simulink subsystem "PvtSubSys_VSM_LCKIE"  (R2020b)
settings: Solver=VariableStepAuto  StartTime=0.0  StopTime=10.0  RelTol=1e-3
values from neighbouring files (symbols this model uses):
  P_VSM_LCKIE_ClassInput = 0.0    [LCKIE.sldd]
  P_VSM_LCKIE_Laneoffset : value not decoded    [LCKIE.sldd]
  P_VSM_LCKIE_Laneoffset_BP : value not decoded    [LCKIE.sldd]
  P_VSM_LCKIE_LatC_DisOffofLanWidth : value not decoded    [LCKIE.sldd]
  P_VSM_LCKIE_LatC_DisOffofSpd : value not decoded    [LCKIE.sldd]
  P_VSM_LCKIE_LatC_DisSW = 0.0    [LCKIE.sldd]
  P_VSM_LCKIE_LatC_LanWidth : value not decoded    [LCKIE.sldd]
  P_VSM_LCKIE_LATC_LimitDis : value not decoded    [LCKIE.sldd]
  P_VSM_LCKIE_LATC_LimitDis_BP : value not decoded    [LCKIE.sldd]
  P_VSM_LCKIE_LatC_LimitDisEgoToObjSelt = 1.5    [LCKIE.sldd]
  P_VSM_LCKIE_LatC_LimitEgoToOppLane = 0.3    [LCKIE.sldd]
  P_VSM_LCKIE_LatC_maxLimitDisREToLane = 2.5    [LCKIE.sldd]
  P_VSM_LCKIE_LatC_minLimitDisREToLane = 1.2    [LCKIE.sldd]
  P_VSM_LCKIE_LatC_MoveEnableDis = 0.0    [LCKIE.sldd]
  P_VSM_LCKIE_LatC_RESafDis = 0.8    [LCKIE.sldd]
  P_VSM_LCKIE_LatC_SafeDisofLanWidth : value not decoded    [LCKIE.sldd]
  P_VSM_LCKIE_LatC_Spd : value not decoded    [LCKIE.sldd]
  P_VSM_LCKIE_LongC_d1 : value not decoded    [LCKIE.sldd]
  P_VSM_LCKIE_LongC_d2 : value not decoded    [LCKIE.sldd]
  P_VSM_LCKIE_LongC_DetaSpd : value not decoded    [LCKIE.sldd]
  P_VSM_LCKIE_LongC_DirecChangeDis = 20.0    [LCKIE.sldd]
  P_VSM_LCKIE_LongC_FleetOff = 80.0    [LCKIE.sldd]
  P_VSM_LCKIE_LongC_maxDis = 80.0    [LCKIE.sldd]
  P_VSM_LCKIE_LongC_minDis = 50.0    [LCKIE.sldd]
  P_VSM_LCKIE_LongC_ShutDownLongDis = -25.0    [LCKIE.sldd]
  P_VSM_LCKIE_LongC_ShutDownTTC = -4.0    [LCKIE.sldd]
  P_VSM_LCKIE_LongC_Spd : value not decoded    [LCKIE.sldd]
  P_VSM_LCKIE_LongC_toff = 10.0    [LCKIE.sldd]
  P_VSM_LCKIE_OFC_ActDis = 10.0    [LCKIE.sldd]
  P_VSM_LCKIE_OFC_DownDis = 10.0    [LCKIE.sldd]
  P_VSM_LCKIE_OFC_DownTTC = 5.0    [LCKIE.sldd]
  P_VSM_LCKIE_OFC_SafDis = 10.0    [LCKIE.sldd]
  P_VSM_LCKIE_OFC_Toff = 3.0    [LCKIE.sldd]
  P_VSM_LCKIE_ORC_LatDis = 1.8    [LCKIE.sldd]
  P_VSM_LCKIE_ORC_LimitDis1 = -30.0    [LCKIE.sldd]
  P_VSM_LCKIE_ORC_LimitDis2 = -10.0    [LCKIE.sldd]
  P_VSM_LCKIE_ORC_LimitTTC = 10.0    [LCKIE.sldd]
  P_VSM_LCKIE_ORC_LowSpd = -5.0    [LCKIE.sldd]
  P_VSM_LCKIE_POC_Delaytime : value not decoded    [LCKIE.sldd]
  P_VSM_LCKIE_POC_detaSpd : value not decoded    [LCKIE.sldd]
  P_VSM_LCKIE_POC_LimitDis = -15.0    [LCKIE.sldd]
  P_VSM_LCKIE_POC_LimitTTC = 2.0    [LCKIE.sldd]
  P_VSM_LCKIE_State_CurveMax = 0.005    [LCKIE.sldd]
  P_VSM_LCKIE_State_CurveMin = 0.0055555555555555558    [LCKIE.sldd]
  P_VSM_LCKIE_State_detaspd = 1.39    [LCKIE.sldd]
  P_VSM_LCKIE_State_detaspd_enable = 1.0    [LCKIE.sldd]
  P_VSM_LCKIE_State_DriverInputTrqValue_enable = 1.0    [LCKIE.sldd]
  P_VSM_LCKIE_State_ELKObjClc = 1.0    [LCKIE.sldd]
  P_VSM_LCKIE_State_HWASts_disable = 1.0    [LCKIE.sldd]
  P_VSM_LCKIE_State_IEObjClc = 1.0    [LCKIE.sldd]
  P_VSM_LCKIE_State_IFVReady = 1.0    [LCKIE.sldd]
  P_VSM_LCKIE_State_lamb_enable = 1.0    [LCKIE.sldd]
  P_VSM_LCKIE_State_Lanecurve_enable = 1.0    [LCKIE.sldd]
  P_VSM_LCKIE_State_LaneWidth_enable = 1.0    [LCKIE.sldd]
  P_VSM_LCKIE_State_Off2on = 3.0    [LCKIE.sldd]
  P_VSM_LCKIE_State_OppObjClc = 1.0    [LCKIE.sldd]
  P_VSM_LCKIE_STATE_ORCObjenable = 0.0    [LCKIE.sldd]
  P_VSM_LCKIE_State_Vehspeed_enable = 1.0    [LCKIE.sldd]
  P_VSM_LCKIE_State_wiper_enable = 1.0    [LCKIE.sldd]
  P_VSM_LCKIE_tcycle = 0.02    [LCKIE.sldd]
undefined symbols (not defined in the file or in its folder): P_Global_Vehicle_Length_m, P_Global_VehicleWidthMin_m, P_VSM_LSMC_SampleTime, STATE
libraries: simulink x62
(part 2 of 5)

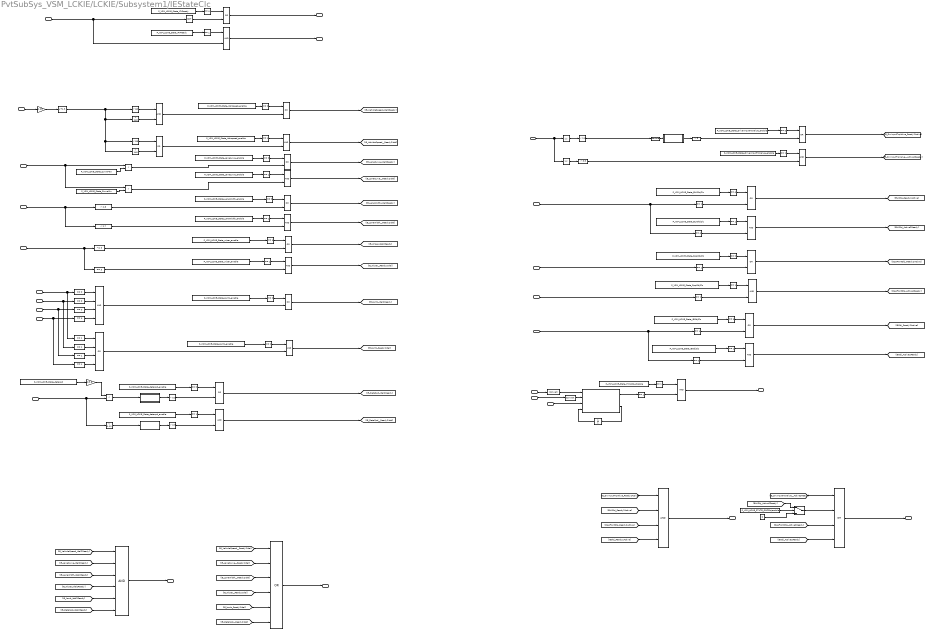
== system PvtSubSys_VSM_LCKIE/LCKIE/Subsystem1/IEStateClc ==
  note: IDEL2READY
  note: READY2ACTIVE
  LaneCurve : Inport
  LaneChange : Inport  Port=2
  OS_Roadwidth : Inport  Port=3
  OS_DetaSpdSelect : Inport  Port=4
  ORC_Clc : Inport  Port=5
  OFC_Ready : Inport  Port=6
  IEObj_Clc : Inport  Port=7
  OFC_Fail : Inport  Port=8
  canABSVehicleSpd : Inport  Port=9
  canBCMWiperSwitchSts : Inport  Port=10
  canBCMHighBeamSts : Inport  Port=11
  canBCMLowBeamSts : Inport  Port=12
  canBCMRearFogLmpSts : Inport  Port=13
  canBCMFrontFogLmpSts : Inport  Port=14
  EPS_DrvInputTrqValue3 : Inport  Port=15
  HWASts : Inport  Port=16
  IFC_Failsafe : Inport  Port=17
  LCKSts : Inport  Port=18
  Abs14 : Abs
  Abs5 : Abs
  Bias : Bias  Bias=1.3
  Compare To Constant1 : simulink/Logic and Bit Operations/Compare To Constant  relop=>  const=60  OutDataTypeStr=boolean
  Compare To Constant{2,7,9..11,14,17..18,23,28..29,33,42..46,48,90,113,182} (21 alike) : simulink/Logic and Bit Operations/Compare To Constant  relop===  const=1  OutDataTypeStr=boolean
  Compare To Constant{8,15..16,19..20,25,30,32,108,124,131..132,137..140,148} (17 alike) : simulink/Logic and Bit Operations/Compare To Constant  relop===  const=0  OutDataTypeStr=boolean
  Compare To Constant111 : simulink/Logic and Bit Operations/Compare To Constant  relop=<  const=55  OutDataTypeStr=boolean
  Compare To Constant112 : simulink/Logic and Bit Operations/Compare To Constant  relop=>  const=145  OutDataTypeStr=boolean
  Compare To Constant12 : simulink/Logic and Bit Operations/Compare To Constant  relop=<  const=-1.12  OutDataTypeStr=boolean
  Compare To Constant13 : simulink/Logic and Bit Operations/Compare To Constant  relop=<  const=2.5  OutDataTypeStr=boolean
  Compare To Constant145 : simulink/Logic and Bit Operations/Compare To Constant  relop=~=  const=3  OutDataTypeStr=boolean
  Compare To Constant21 : simulink/Logic and Bit Operations/Compare To Constant  relop=<  const=140  OutDataTypeStr=boolean
  Compare To Constant24 : simulink/Logic and Bit Operations/Compare To Constant  relop=>  const=0.5  OutDataTypeStr=boolean
  Compare To Constant26 : simulink/Logic and Bit Operations/Compare To Constant  relop=>  const=2.8  OutDataTypeStr=boolean
  Compare To Constant27 : simulink/Logic and Bit Operations/Compare To Constant  relop=<  const=2.7  OutDataTypeStr=boolean
  Compare To Constant3 : simulink/Logic and Bit Operations/Compare To Constant  relop=>  const=0.5  OutDataTypeStr=boolean
  Compare To Constant47 : simulink/Logic and Bit Operations/Compare To Constant  relop===  const=3  OutDataTypeStr=boolean
  Compare To Constant91 : simulink/Logic and Bit Operations/Compare To Constant  relop=>  const=3.5  OutDataTypeStr=boolean
  Compare To Constant31 : simulink/Logic and Bit Operations/Compare To Constant  relop=>  const=3  OutDataTypeStr=boolean
  Constant : Constant  Value=P_VSM_LCKIE_State_CurveMax
  Constant1 : Constant  Value=P_VSM_LCKIE_State_CurveMin
  Constant14 : Constant  Value=P_VSM_LCKIE_State_OppObjClc
  Constant15 : Constant  Value=P_VSM_LCKIE_State_IEObjClc
  Constant2 : Constant  Value=P_VSM_LCKIE_State_ELKObjClc
  Constant3 : Constant  Value=P_VSM_LCKIE_STATE_ORCObjenable
  Constant4 : Constant  Value=P_VSM_LCKIE_State_IEObjClc
  Constant5 : Constant  Value=0  OutDataTypeStr=boolean
  Constant8 : Constant  Value=P_VSM_LCKIE_State_ELKObjClc
  Constant9 : Constant  Value=P_VSM_LCKIE_State_OppObjClc
  Data Type Conversion : DataTypeConversion
  Data Type Conversion1 : DataTypeConversion
  Data Type Conversion15 : DataTypeConversion  OutDataTypeStr=double
  Gain : Gain  Gain=1/3.6
  Gain2 : Gain  Gain=1.03
  Logical Operator{1,4..5,9,11..13,17..18,21,49,60,64} (13 alike) : Logic  AllPortsSameDT=off  OutDataTypeStr=boolean
  Logical Operator{6..8,10,20,36,57,59,69,82..83,109} (12 alike) : Logic  Operator=OR  AllPortsSameDT=off  OutDataTypeStr=boolean
  Logical Operator101 : Logic  Operator=NOT  AllPortsSameDT=off  OutDataTypeStr=boolean
  Logical Operator14 : Logic  Inputs=6  AllPortsSameDT=off  OutDataTypeStr=boolean
  Logical Operator15 : Logic  Operator=OR  Inputs=6  AllPortsSameDT=off  OutDataTypeStr=boolean
  Logical Operator16 : Logic  Inputs=4  AllPortsSameDT=off  OutDataTypeStr=boolean
  Logical Operator19 : Logic  Operator=OR  Inputs=4  AllPortsSameDT=off  OutDataTypeStr=boolean
  Logical Operator22 : Logic  Operator=OR  Inputs=4  AllPortsSameDT=off  OutDataTypeStr=boolean
  Logical Operator89 : Logic  Inputs=4  AllPortsSameDT=off  OutDataTypeStr=boolean
  MATLAB Function1 : MATLAB Function  TreatAsAtomicUnit=on
  Relational Operator : RelationalOperator  Operator=<  OutDataTypeStr=boolean  RndMeth=Simplest
  Relational Operator1 : RelationalOperator  Operator=<  OutDataTypeStr=boolean  RndMeth=Simplest
  Relational Operator2 : RelationalOperator  Operator=>  OutDataTypeStr=boolean  RndMeth=Simplest
  Subsystem1 : Subsystem  mask{Ts=P_VSM_LSMC_SampleTime, Max=10}
      mask prompts: Ts "Sample Time:"; Max "Max Limit:"
      mask Display:
      | Ts=get_param(gcb,'Ts');
      | Max=get_param(gcb,'Max');
      | disp(['Ts:' Ts '\n' 'Max:' Max ]);
  Subsystem12 : Subsystem  mask{Ts=P_VSM_LSMC_SampleTime, Max=10}
      mask prompts: Ts "Sample Time:"; Max "Max Limit:"
      mask Display:
      | Ts=get_param(gcb,'Ts');
      | Max=get_param(gcb,'Max');
      | disp(['Ts:' Ts '\n' 'Max:' Max ]);
  Subsystem4 : Subsystem  mask{Ts=P_VSM_LSMC_SampleTime, Max=10}
      mask prompts: Ts "Sample Time:"; Max "Max Limit:"
      mask Display:
      | Ts=get_param(gcb,'Ts');
      | Max=get_param(gcb,'Max');
      | disp(['Ts:' Ts '\n' 'Max:' Max ]);
  Switch : Switch  Criteria=u2 > Threshold
  Unit Delay2 : UnitDelay  SampleTime=-1  HasFrameUpgradeWarning=on
  param_1 : Constant  Value=P_VSM_LCKIE_State_detaspd_enable
  param_14 : Constant  Value=P_VSM_LCKIE_State_wiper_enable
  param_15 : Constant  Value=P_VSM_LCKIE_State_lamb_enable
  param_16 : Constant  Value=P_VSM_LCKIE_State_Lanecurve_enable
  param_17 : Constant  Value=P_VSM_LCKIE_State_LaneWidth_enable
  param_2 : Constant  Value=P_VSM_LCKIE_State_detaspd_enable
  param_3 : Constant  Value=P_VSM_LCKIE_State_HWASts_disable
  param_31 : Constant  Value=P_VSM_LCKIE_State_Vehspeed_enable
  param_35 : Constant  Value=P_VSM_LCKIE_State_DriverInputTrqValue_enable
  param_4 : Constant  Value=P_VSM_LCKIE_State_Vehspeed_enable
  param_40 : Constant  Value=P_VSM_LCKIE_State_LaneWidth_enable
  param_45 : Constant  Value=P_VSM_LCKIE_State_wiper_enable
  param_46 : Constant  Value=P_VSM_LCKIE_State_lamb_enable
  param_5 : Constant  Value=P_VSM_LCKIE_State_detaspd
  param_6 : Constant  Value=P_VSM_LCKIE_State_IFVReady
  param_67 : Constant  Value=P_VSM_LCKIE_State_IFVReady
  param_7 : Constant  Value=P_VSM_LCKIE_State_DriverInputTrqValue_enable
  param_9 : Constant  Value=P_VSM_LCKIE_State_Lanecurve_enable
  IFVReady : Outport
  IFVFail : Outport  Port=2
  IE_Idel2Ready : Outport  Port=3
  IE_Ready2Idel : Outport  Port=4
  IE__Ready2Active : Outport  Port=5
  IE__Active2Ready : Outport  Port=6
  HWAReady : Outport  Port=7
  wires:
  [ELKObj_Active2Ready] -> Switch/1
  [OppFrontObj_Active2Ready] -> Logical Operator22/3
  [IEObj_Active2Ready] -> Logical Operator22/4
  [IE_DrvInputTrqValue__Active2Ready] -> Logical Operator22/1
  Logical Operator22/1 -> IE__Active2Ready/1  "VSM_LCKIE_State_Active2Ready"
  Logical Operator16/1 -> IE__Ready2Active/1  "VSM_LCKIE_State_Ready2Active"
  [IEObj_Ready2Active] -> Logical Operator16/4
  [OppFrontObj_Ready2Active] -> Logical Operator16/3
  [ELKObj_Ready2Active] -> Logical Operator16/2
  [IE_DrvInputTrqValue_Ready2Active] -> Logical Operator16/1
  Logical Operator15/1 -> IE_Ready2Idel/1  "VSM_LCKIE_State_Ready2Idel"
  [IE_DetaSpd__Ready2Idel] -> Logical Operator15/6
  [IE_lamb_Ready2Idel] -> Logical Operator15/5
  [IE_Wiper__Ready2Idel] -> Logical Operator15/4
  [IE_LaneWidth__Ready2Idel] -> Logical Operator15/3
  [IE_LaneCurve__Ready2Idel] -> Logical Operator15/2
  [IE_VehicleSpeed__Ready2Idel] -> Logical Operator15/1
  Logical Operator14/1 -> IE_Idel2Ready/1  "VSM_LCKIE_State_Idel2Ready"
  [IE_DetaSpd_Idel2Ready] -> Logical Operator14/6
  [IE_lamb_Idel2Ready] -> Logical Operator14/5
  [IE_Wiper_Idel2Ready] -> Logical Operator14/4
  [IE_LaneWidth_Idel2Ready] -> Logical Operator14/3
  [IE_LaneCurve_Idel2Ready] -> Logical Operator14/2
  [IE_VehicleSpeed_Idel2Ready] -> Logical Operator14/1
  Gain/1 -> Relational Operator/1
  param_5/1 -> Gain/1
  OFC_Fail/1 -> Compare To Constant11/1
  Compare To Constant9/1 -> Logical Operator12/1
  Constant8/1 -> Compare To Constant33/1
  Constant4/1 -> Compare To Constant16/1
  Logical Operator6/1 -> [ELKObj_Ready2Active]  "VSM_LCKIE_State_ELKObj_Ready2Active"
  Logical Operator10/1 -> [OppFrontObj_Ready2Active]  "VSM_LCKIE_State_OppFrontObj_Ready2Active"
  Compare To Constant18/1 -> Logical Operator6/2
  Constant15/1 -> Compare To Constant17/1
  IEObj_Clc/1 -> Compare To Constant29/1, Compare To Constant30/1
  Constant9/1 -> Compare To Constant9/1
  Logical Operator7/1 -> [IEObj_Ready2Active]  "VSM_LCKIE_State_IEObj_Ready2Active"
  Logical Operator13/1 -> [IEObj_Active2Ready]  "VSM_LCKIE_State_IEObj_Active2Ready"
  Compare To Constant8/1 -> Logical Operator10/1
  Compare To Constant11/1 -> Logical Operator12/2
  ORC_Clc/1 -> Compare To Constant18/1, Compare To Constant19/1
  Compare To Constant10/1 -> Logical Operator10/2
  Compare To Constant32/1 -> Logical Operator6/1
  Compare To Constant19/1 -> Logical Operator9/2
  Constant2/1 -> Compare To Constant32/1
  Compare To Constant30/1 -> Logical Operator13/2
  Compare To Constant29/1 -> Logical Operator7/2
  Compare To Constant16/1 -> Logical Operator7/1
  Compare To Constant17/1 -> Logical Operator13/1
  Logical Operator12/1 -> [OppFrontObj_Active2Ready]  "VSM_LCKIE_State_OppFrontObj_Active2Ready"
  OFC_Ready/1 -> Compare To Constant10/1
  Constant14/1 -> Compare To Constant8/1
  Logical Operator9/1 -> [ELKObj_Active2Ready]  "VSM_LCKIE_State_ELKObj_Active2Ready"
  Compare To Constant33/1 -> Logical Operator9/1
  IFC_Failsafe/1 -> Logical Operator101/1, Logical Operator5/2
  Compare To Constant148/1 -> Logical Operator109/1
  Logical Operator5/1 -> IFVFail/1  "VSM_LCKIE_State_IFVFail"
  Logical Operator109/1 -> IFVReady/1  "VSM_LCKIE_State_IFVReady"
  param_67/1 -> Compare To Constant182/1
  param_6/1 -> Compare To Constant148/1
  Compare To Constant182/1 -> Logical Operator5/1
  Logical Operator101/1 -> Logical Operator109/2
  Data Type Conversion15/1 -> Subsystem12/1(In1)
  Compare To Constant90/1 -> Logical Operator49/1
  Compare To Constant124/1 -> Logical Operator69/1
  EPS_DrvInputTrqValue3/1 -> Abs5/1, Abs14/1
  Compare To Constant13/1 -> Data Type Conversion15/1
  Compare To Constant31/1 -> Logical Operator69/2
  Abs14/1 -> Compare To Constant91/1
  Logical Operator49/1 -> [IE_DrvInputTrqValue__Active2Ready]  "VSM_LCKIE_State_DrvInputTrqValue_Active2Ready"
  Subsystem12/1(Out1) -> Compare To Constant31/1
  Logical Operator69/1 -> [IE_DrvInputTrqValue_Ready2Active]  "VSM_LCKIE_State_DrvInputTrqValue_Ready2Active"
  Abs5/1 -> Compare To Constant13/1
  param_35/1 -> Compare To Constant90/1
  Compare To Constant91/1 -> Logical Operator49/2
  param_7/1 -> Compare To Constant124/1
  HWASts/1 -> Data Type Conversion/1
  param_3/1 -> Compare To Constant7/1
  Compare To Constant7/1 -> Logical Operator4/1
  Logical Operator4/1 -> HWAReady/1  "VSM_LCKIE_State_HWASts_Ready2Active"
  Logical Operator1/1 -> [IE_DetaSpd__Ready2Idel]  "VSM_LCKIE_State_detaspd_Ready2Idel"
  Compare To Constant12/1 -> Subsystem4/1(In1)
  Compare To Constant2/1 -> Logical Operator1/1
  param_2/1 -> Compare To Constant2/1
  Compare To Constant3/1 -> Logical Operator1/2
  Subsystem4/1(Out1) -> Compare To Constant3/1
  Subsystem1/1(Out1) -> Compare To Constant24/1
  Compare To Constant24/1 -> Logical Operator8/2
  param_1/1 -> Compare To Constant15/1
  Relational Operator/1 -> Subsystem1/1(In1)
  Logical Operator8/1 -> [IE_DetaSpd_Idel2Ready]  "VSM_LCKIE_State_detaspd_Idel2Ready"
  Compare To Constant15/1 -> Logical Operator8/1
  OS_DetaSpdSelect/1 -> Compare To Constant12/1, Relational Operator/2
  Compare To Constant131/1 -> Logical Operator82/1
  param_45/1 -> Compare To Constant131/1
  Logical Operator83/1 -> [IE_lamb_Idel2Ready]  "VSM_LCKIE_State_lamb_Idel2Ready"
  Compare To Constant139/1 -> Logical Operator89/3
  Logical Operator82/1 -> [IE_Wiper_Idel2Ready]  "VSM_LCKIE_State_wiper_Idel2Ready"
  canBCMLowBeamSts/1 -> Compare To Constant138/1, Compare To Constant44/1
  canBCMWiperSwitchSts/1 -> Compare To Constant145/1, Compare To Constant47/1
  canBCMHighBeamSts/1 -> Compare To Constant137/1, Compare To Constant42/1
  param_46/1 -> Compare To Constant132/1
  Logical Operator89/1 -> Logical Operator83/2
  Compare To Constant137/1 -> Logical Operator89/1
  canBCMFrontFogLmpSts/1 -> Compare To Constant140/1, Compare To Constant46/1
  Compare To Constant140/1 -> Logical Operator89/4
  Compare To Constant145/1 -> Logical Operator82/2
  Compare To Constant132/1 -> Logical Operator83/1
  canBCMRearFogLmpSts/1 -> Compare To Constant139/1, Compare To Constant45/1
  Compare To Constant138/1 -> Logical Operator89/2
  Compare To Constant27/1 -> Logical Operator21/2
  Logical Operator21/1 -> [IE_LaneWidth__Ready2Idel]  "VSM_LCKIE_State_LaneWidth_Ready2Idel"
  Compare To Constant28/1 -> Logical Operator21/1
  param_17/1 -> Compare To Constant28/1
  Compare To Constant26/1 -> Logical Operator20/2
  param_40/1 -> Compare To Constant25/1
  Logical Operator20/1 -> [IE_LaneWidth_Idel2Ready]  "VSM_LCKIE_State_LaneWidth_Idel2Ready"
  Compare To Constant25/1 -> Logical Operator20/1
  OS_Roadwidth/1 -> Compare To Constant26/1, Compare To Constant27/1
  Compare To Constant23/1 -> Logical Operator11/1
  Relational Operator2/1 -> Logical Operator11/2
  param_16/1 -> Compare To Constant23/1
  Logical Operator11/1 -> [IE_LaneCurve__Ready2Idel]  "VSM_LCKIE_State_Lanecurve_Ready2Idel"
  Logical Operator36/1 -> [IE_LaneCurve_Idel2Ready]  "VSM_LCKIE_State_Lanecurve_Idel2Ready"
  param_9/1 -> Compare To Constant108/1
  LaneCurve/1 -> Relational Operator2/1, Relational Operator1/1
  Relational Operator1/1 -> Logical Operator36/2
  Compare To Constant108/1 -> Logical Operator36/1
  Compare To Constant21/1 -> Logical Operator60/2
  Bias/1 -> Compare To Constant112/1, Compare To Constant111/1, Compare To Constant21/1, Compare To Constant1/1
  param_31/1 -> Compare To Constant20/1
  param_4/1 -> Compare To Constant113/1
  Compare To Constant112/1 -> Logical Operator57/2
  Logical Operator59/1 -> [IE_VehicleSpeed_Idel2Ready]  "VSM_LCKIE_State_Vehspeed_Idel2Ready"
  Logical Operator57/1 -> Logical Operator64/2
  Logical Operator64/1 -> [IE_VehicleSpeed__Ready2Idel]  "VSM_LCKIE_State_Vehspeed_Ready2Idel"
  Compare To Constant20/1 -> Logical Operator59/1
  Compare To Constant113/1 -> Logical Operator64/1
  Gain2/1 -> Bias/1
  canABSVehicleSpd/1 -> Gain2/1
  Compare To Constant1/1 -> Logical Operator60/1
  Logical Operator60/1 -> Logical Operator59/2
  Compare To Constant111/1 -> Logical Operator57/1
  Compare To Constant45/1 -> Logical Operator19/3
  param_15/1 -> Compare To Constant43/1
  Compare To Constant42/1 -> Logical Operator19/1
  Logical Operator17/1 -> [IE_lamb_Ready2Idel]  "VSM_LCKIE_State_lamb_Ready2Idel"
  Compare To Constant47/1 -> Logical Operator18/2
  Logical Operator18/1 -> [IE_Wiper__Ready2Idel]  "VSM_LCKIE_State_wiper_Ready2Idel"
  Compare To Constant44/1 -> Logical Operator19/2
  Logical Operator19/1 -> Logical Operator17/2
  Compare To Constant43/1 -> Logical Operator17/1
  Compare To Constant48/1 -> Logical Operator18/1
  Compare To Constant46/1 -> Logical Operator19/4
  param_14/1 -> Compare To Constant48/1
  Unit Delay2/1 -> MATLAB Function1/4(reflgK1)
  LaneChange/1 -> MATLAB Function1/3(LaneChange)
  MATLAB Function1/1(Flg) -> Compare To Constant14/1
  MATLAB Function1/2(reflg) -> Unit Delay2/1
  Data Type Conversion/1 -> MATLAB Function1/1(HWASts)
  Compare To Constant14/1 -> Logical Operator4/2
  LCKSts/1 -> Data Type Conversion1/1
  Data Type Conversion1/1 -> MATLAB Function1/2(LCKSts)
  Constant/1 -> Relational Operator1/2
  Constant1/1 -> Relational Operator2/2
  Switch/1 -> Logical Operator22/2
  Constant3/1 -> Switch/2
  Constant5/1 -> Switch/3

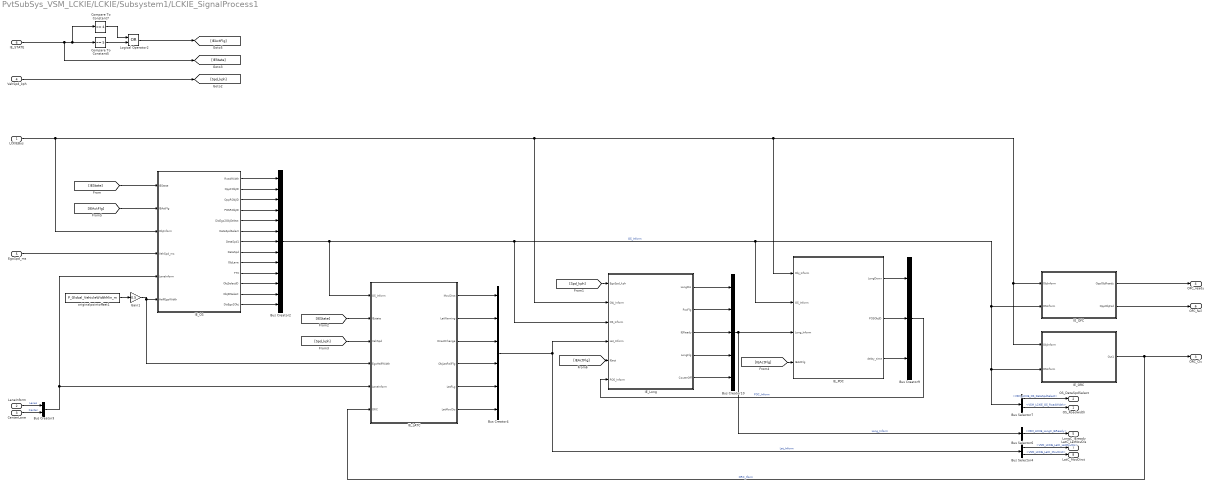
== system PvtSubSys_VSM_LCKIE/LCKIE/Subsystem1/LCKIE_SignalProcess1 ==
  LCKIEBus : Inport
  LaneInform : Inport  Port=2
  CenterLane : Inport  Port=3
  VehSpd_kph : Inport  Port=4  OutDataTypeStr=single
  EgoSpd_ms : Inport  Port=5
  IE_STATE : Inport  Port=6
  Bus Creator10 : BusCreator  Inputs=5
  Bus Creator2 : BusCreator  Inputs=13
  Bus Creator3 : BusCreator  Inputs=2
  Bus Creator4 : BusCreator  Inputs=6
  Bus Creator9 : BusCreator  Inputs=3
  Bus Selector4 : BusSelector  OutputSignals=VSM_LCKIE_LatC_LatMovDis,VSM_LCKIE_LatC_MovDirct
  Bus Selector6 : BusSelector  OutputSignals=VSM_LCKIE_LongC_IEReady
  Bus Selector7 : BusSelector  OutputSignals=VSM_LCKIE_OS_DetaSpdSelect,VSM_LCKIE_OS_RoadWidth
  Compare To Constant5 : simulink/Logic and Bit Operations/Compare To Constant  relop===  const=5  OutDataTypeStr=boolean
  Compare To Constant7 : simulink/Logic and Bit Operations/Compare To Constant  relop===  const=4  OutDataTypeStr=boolean
  Gain1 : Gain  Gain=0.5  OutDataTypeStr=single
  IE_LATC : Subsystem
  IE_Long : Subsystem
  IE_OFC : Subsystem
  IE_ORC : Subsystem
  IE_OS : Subsystem
  IE_POC : Subsystem
  Logical Operator2 : Logic  Operator=OR  AllPortsSameDT=off  OutDataTypeStr=boolean
  originalpointoffset1 : Constant  Value=P_Global_VehicleWidthMin_m
  OS_Roadwidth : Outport
  OS_DetaSpdSelect : Outport  Port=2
  ORC_Clc : Outport  Port=3
  OFC_ready : Outport  Port=4
  LongC_IEready : Outport  Port=5
  OFC_fail : Outport  Port=6
  LatC_LatMovDis : Outport  Port=7
  LatC_MovDirct : Outport  Port=8
  wires:
  IE_ORC/1(Out1) -> ORC_Clc/1, IE_LATC/6(ORC)  "ORC_Iform"
  IE_POC/2(POSObjID) -> Bus Creator9/2
  IE_POC/1(LongDown) -> Bus Creator9/1
  [IEActFlg] -> IE_POC/4(IEActFlg)
  IE_LATC/1(MovDirct) -> Bus Creator4/1
  IE_STATE/1 -> Compare To Constant7/1, Compare To Constant5/1, [IEState]
  IE_OS/1(RoadWidth) -> Bus Creator2/1
  IE_OS/11(ObjSelectID) -> Bus Creator2/11
  IE_OS/6(DetaSpdSelect) -> Bus Creator2/6
  [IEState] -> IE_OS/1(IEState)
  IE_OFC/2(OppObjFail) -> OFC_fail/1
  Bus Creator3/1 -> IE_LATC/5(LaneInform), IE_OS/5(LaneInform)
  IE_OS/4(POSRObjID) -> Bus Creator2/4
  IE_LATC/5(LatFLg) -> Bus Creator4/5
  Bus Selector4/2 -> LatC_MovDirct/1  "<VSM_LCKIE_LatC_MovDirct>"
  Bus Selector4/1 -> LatC_LatMovDis/1  "<VSM_LCKIE_LatC_LatMovDis>"
  IE_OS/12(ObjIDSelect) -> Bus Creator2/12
  IE_Long/1(LongDis) -> Bus Creator10/1
  IE_LATC/2(LatWarning) -> Bus Creator4/2
  Bus Selector6/1 -> LongC_IEready/1  "<VSM_LCKIE_LongC_IEReady>"
  IE_OS/7(DetaSpd1) -> Bus Creator2/7
  Gain1/1 -> IE_OS/6(HalfEgoWidth), IE_LATC/4(EgoHalfWidth)
  IE_Long/3(IEReady) -> Bus Creator10/3
  VehSpd_kph/1 -> [Spd_kph]
  Bus Creator4/1 -> IE_Long/4(Lat_Inform), Bus Selector4/1  "Lat_Inform"
  IE_LATC/6(LatMovDis) -> Bus Creator4/6
  CenterLane/1 -> Bus Creator3/2  "Center"
  IE_Long/4(LongFlg) -> Bus Creator10/4
  Bus Selector7/2 -> OS_Roadwidth/1  "<VSM_LCKIE_OS_RoadWidth>"
  LaneInform/1 -> Bus Creator3/1  "Lanes"
  IE_OS/8(DetaSpd) -> Bus Creator2/8
  [Spd_kph] -> IE_LATC/3(VehSpd)
  IE_OS/5(DisEgo2ObjSelect) -> Bus Creator2/5
  IE_Long/2(PocFlg) -> Bus Creator10/2
  IE_OS/3(OppRObjID) -> Bus Creator2/3
  Bus Selector7/1 -> OS_DetaSpdSelect/1  "<VSM_LCKIE_OS_DetaSpdSelect>"
  [IEState] -> IE_LATC/2(IEstate)
  IE_POC/3(delay_time) -> Bus Creator9/3
  EgoSpd_ms/1 -> IE_OS/4(VehSpd_ms)
  LCKIEBus/1 -> IE_OS/3(ObjInform), IE_POC/1(Obj_Inform), IE_ORC/1(ObjInform), IE_OFC/1(ObjInform), IE_Long/2(Obj_Inform)
  IE_OS/10(TTC) -> Bus Creator2/10
  Logical Operator2/1 -> [IEActFlg]
  IE_Long/5(CouterOff) -> Bus Creator10/5
  Bus Creator9/1 -> IE_Long/6(POS_Inform)  "POC_Inform"
  [Spd_kph] -> IE_Long/1(EgoSpd_kph)
  Compare To Constant7/1 -> Logical Operator2/1
  IE_OS/9(ObjLane) -> Bus Creator2/9
  IE_OFC/1(OppObjReady) -> OFC_ready/1
  IE_LATC/3(DirectChange) -> Bus Creator4/3
  Bus Creator2/1 -> IE_POC/2(OS_Inform), IE_ORC/2(OSInform), Bus Selector7/1, IE_OFC/2(OSInform), IE_Long/3(OS_Inform), IE_LATC/1(OS_Inform)  "OS_Inform"
  [IEActFlg] -> IE_OS/2(IEActFlg)
  Bus Creator10/1 -> Bus Selector6/1, IE_POC/3(Long_Inform)  "Long_Inform"
  IE_OS/2(OppFObjID) -> Bus Creator2/2
  IE_LATC/4(ObjLatFailFlg) -> Bus Creator4/4
  Compare To Constant5/1 -> Logical Operator2/2
  originalpointoffset1/1 -> Gain1/1
  IE_OS/13(DisEgo2Obj) -> Bus Creator2/13
  [IEActFlg] -> IE_Long/5(IEact)

== system PvtSubSys_VSM_LCKIE/LCKIE/Subsystem1/IEStateClc/Subsystem1 ==
  In1 : Inport
  Add : Sum
  Constant : Constant  Value=Ts
  Constant1 : Constant  Value=0
  Constant2 : Constant  Value=Max
  Max : MinMax  Inputs=2
  Switch : Switch  Criteria=u2 ~= 0
  Unit Delay : UnitDelay  SampleTime=-1  HasFrameUpgradeWarning=on
  Out1 : Outport
  wires:
  Switch/1 -> Max/1
  Constant2/1 -> Max/2
  Max/1 -> Out1/1, Unit Delay/1
  Add/1 -> Switch/1
  Constant1/1 -> Switch/3
  Constant/1 -> Add/2
  In1/1 -> Switch/2
  Unit Delay/1 -> Add/1

== system PvtSubSys_VSM_LCKIE/LCKIE/Subsystem1/IEStateClc/Subsystem12 ==
  In1 : Inport
  Add : Sum
  Constant : Constant  Value=Ts
  Constant1 : Constant  Value=0
  Constant2 : Constant  Value=Max
  Max : MinMax  Inputs=2
  Switch : Switch  Criteria=u2 ~= 0
  Unit Delay : UnitDelay  SampleTime=-1  HasFrameUpgradeWarning=on
  Out1 : Outport
  wires:
  Unit Delay/1 -> Add/1
  In1/1 -> Switch/2
  Constant/1 -> Add/2
  Constant1/1 -> Switch/3
  Add/1 -> Switch/1
  Max/1 -> Unit Delay/1, Out1/1
  Constant2/1 -> Max/2
  Switch/1 -> Max/1

== system PvtSubSys_VSM_LCKIE/LCKIE/Subsystem1/IEStateClc/Subsystem4 ==
  In1 : Inport
  Add : Sum
  Constant : Constant  Value=Ts
  Constant1 : Constant  Value=0
  Constant2 : Constant  Value=Max
  Max : MinMax  Inputs=2
  Switch : Switch  Criteria=u2 ~= 0
  Unit Delay : UnitDelay  SampleTime=-1  HasFrameUpgradeWarning=on
  Out1 : Outport
  wires:
  Unit Delay/1 -> Add/1
  In1/1 -> Switch/2
  Constant/1 -> Add/2
  Constant1/1 -> Switch/3
  Add/1 -> Switch/1
  Max/1 -> Unit Delay/1, Out1/1
  Constant2/1 -> Max/2
  Switch/1 -> Max/1
